simulink model "Blood_platelet_Count_V3"  (R2022a)
settings: Solver=VariableStepAuto  StartTime=0.0  StopTime=10.0  RelTol=1e-3
libraries: simulink x9
settings Model: Creator=KVJ RAMAN  LastModifiedBy=hp

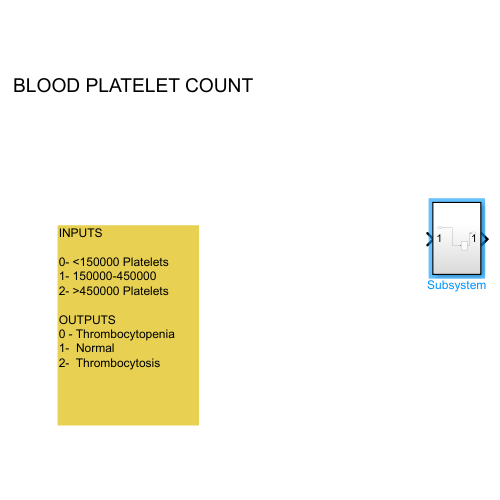
[thumbnail: Simulink's stored preview of the top-level diagram]
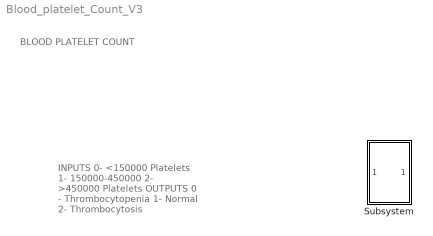
== system Blood_platelet_Count_V3 ==
  note: BLOOD PLATELET COUNT
  note: INPUTS
      |
      | 0- <150000 Platelets
      | 1- 150000-450000
      | 2- >450000 Platelets
      |
      | OUTPUTS
      | 0 - Thrombocytopenia
      | 1-  Normal
      | 2-  Thrombocytosis
  Subsystem : Subsystem

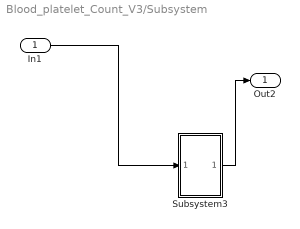
== system Blood_platelet_Count_V3/Subsystem ==
  In1 : Inport
  Subsystem3 : Subsystem
  Out2 : Outport
  wires:
  In1/1 -> Subsystem3/1(In1)
  Subsystem3/1(Out2) -> Out2/1

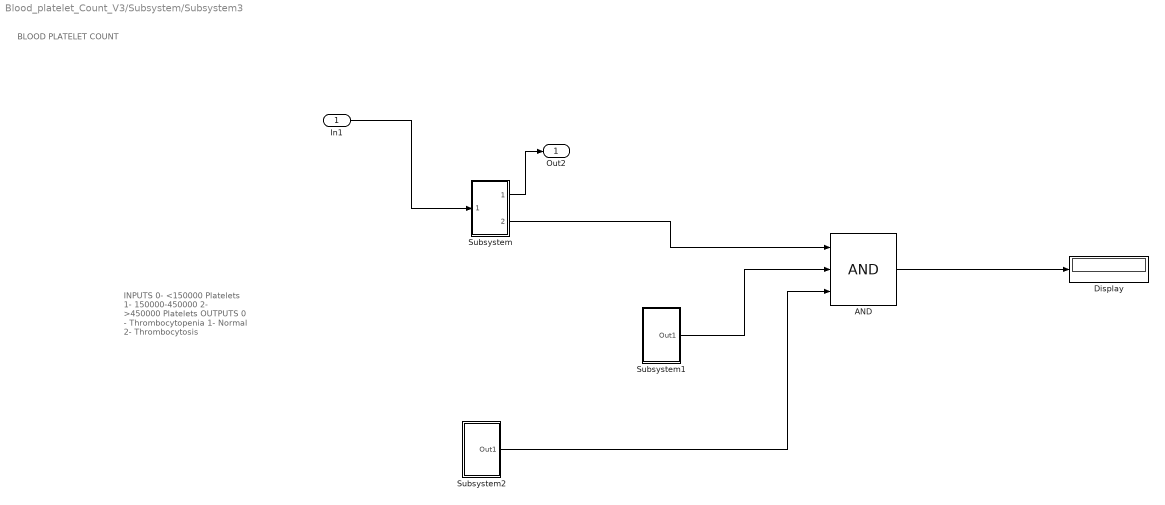
== system Blood_platelet_Count_V3/Subsystem/Subsystem3 ==
  note: BLOOD PLATELET COUNT
  note: INPUTS
      |
      | 0- <150000 Platelets
      | 1- 150000-450000
      | 2- >450000 Platelets
      |
      | OUTPUTS
      | 0 - Thrombocytopenia
      | 1-  Normal
      | 2-  Thrombocytosis
  In1 : Inport
  AND : Logic  Inputs=3  IconShape=distinctive  AllPortsSameDT=off  OutDataTypeStr=boolean
  Display : Display
  Subsystem : Subsystem
  Subsystem1 : Subsystem
  Subsystem2 : Subsystem
  Out2 : Outport
  wires:
  Subsystem2/1(Out1) -> AND/3
  AND/1 -> Display/1
  Subsystem/1(Out2) -> Out2/1
  Subsystem/2(Out1) -> AND/1
  Subsystem1/1(Out1) -> AND/2
  In1/1 -> Subsystem/1(In1)

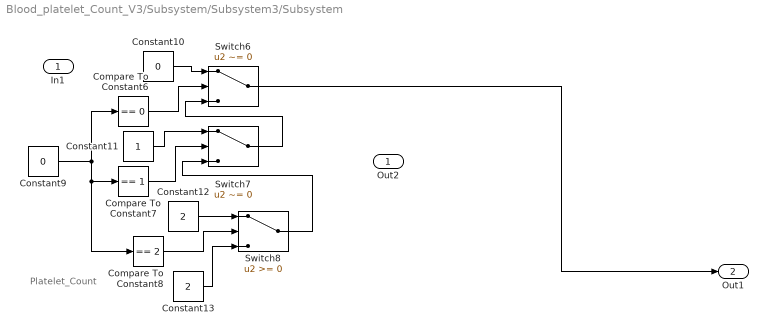
== system Blood_platelet_Count_V3/Subsystem/Subsystem3/Subsystem ==
  note: Platelet_Count
  In1 : Inport
  Compare To Constant6 : simulink/Logic and Bit Operations/Compare To Constant  relop===  const=0  OutDataTypeStr=boolean
  Compare To Constant7 : simulink/Logic and Bit Operations/Compare To Constant  relop===  const=1  OutDataTypeStr=boolean
  Compare To Constant8 : simulink/Logic and Bit Operations/Compare To Constant  relop===  const=2  OutDataTypeStr=boolean
  Constant10 : Constant  Value=0
  Constant11 : Constant
  Constant12 : Constant  Value=2
  Constant13 : Constant  Value=2
  Constant9 : Constant  Value=0
  Switch6 : Switch  Criteria=u2 ~= 0  SaturateOnIntegerOverflow=off  InputSameDT=off
  Switch7 : Switch  Criteria=u2 ~= 0  SaturateOnIntegerOverflow=off  InputSameDT=off
  Switch8 : Switch  SaturateOnIntegerOverflow=off  InputSameDT=off
  Out2 : Outport
  Out1 : Outport  Port=2
  wires:
  Constant11/1 -> Switch7/1
  Compare To Constant6/1 -> Switch6/2
  Switch6/1 -> Out1/1
  Constant9/1 -> Compare To Constant6/1, Compare To Constant8/1, Compare To Constant7/1
  Switch8/1 -> Switch7/3
  Constant10/1 -> Switch6/1
  Compare To Constant7/1 -> Switch7/2
  Switch7/1 -> Switch6/3
  Constant13/1 -> Switch8/3
  Constant12/1 -> Switch8/1
  Compare To Constant8/1 -> Switch8/2

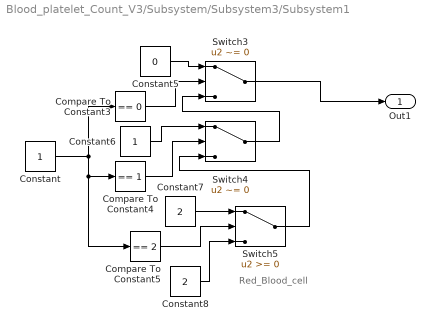
== system Blood_platelet_Count_V3/Subsystem/Subsystem3/Subsystem1 ==
  note: Red_Blood_cell
  Compare To Constant3 : simulink/Logic and Bit Operations/Compare To Constant  relop===  const=0  OutDataTypeStr=boolean
  Compare To Constant4 : simulink/Logic and Bit Operations/Compare To Constant  relop===  const=1  OutDataTypeStr=boolean
  Compare To Constant5 : simulink/Logic and Bit Operations/Compare To Constant  relop===  const=2  OutDataTypeStr=boolean
  Constant : Constant
  Constant5 : Constant  Value=0
  Constant6 : Constant
  Constant7 : Constant  Value=2
  Constant8 : Constant  Value=2
  Switch3 : Switch  Criteria=u2 ~= 0  SaturateOnIntegerOverflow=off  InputSameDT=off
  Switch4 : Switch  Criteria=u2 ~= 0  SaturateOnIntegerOverflow=off  InputSameDT=off
  Switch5 : Switch  SaturateOnIntegerOverflow=off  InputSameDT=off
  Out1 : Outport
  wires:
  Switch4/1 -> Switch3/3
  Compare To Constant4/1 -> Switch4/2
  Constant6/1 -> Switch4/1
  Switch5/1 -> Switch4/3
  Constant5/1 -> Switch3/1
  Constant8/1 -> Switch5/3
  Compare To Constant5/1 -> Switch5/2
  Constant7/1 -> Switch5/1
  Compare To Constant3/1 -> Switch3/2
  Constant/1 -> Compare To Constant3/1, Compare To Constant5/1, Compare To Constant4/1
  Switch3/1 -> Out1/1

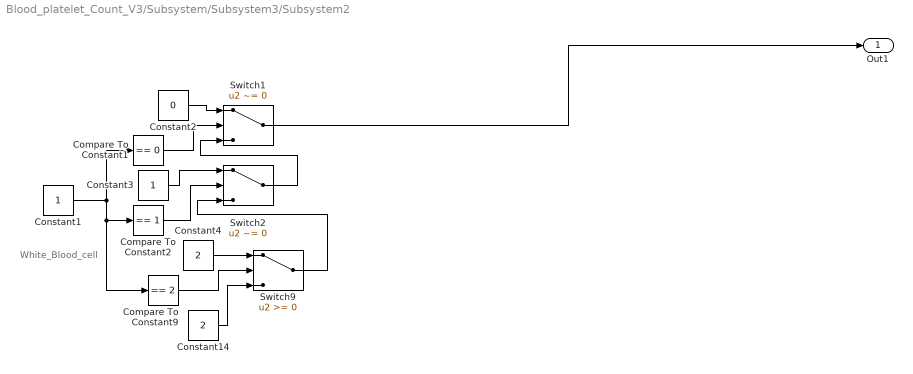
== system Blood_platelet_Count_V3/Subsystem/Subsystem3/Subsystem2 ==
  note: White_Blood_cell
  Compare To Constant1 : simulink/Logic and Bit Operations/Compare To Constant  relop===  const=0  OutDataTypeStr=boolean
  Compare To Constant2 : simulink/Logic and Bit Operations/Compare To Constant  relop===  const=1  OutDataTypeStr=boolean
  Compare To Constant9 : simulink/Logic and Bit Operations/Compare To Constant  relop===  const=2  OutDataTypeStr=boolean
  Constant1 : Constant
  Constant14 : Constant  Value=2
  Constant2 : Constant  Value=0
  Constant3 : Constant
  Constant4 : Constant  Value=2
  Switch1 : Switch  Criteria=u2 ~= 0  SaturateOnIntegerOverflow=off  InputSameDT=off
  Switch2 : Switch  Criteria=u2 ~= 0  SaturateOnIntegerOverflow=off  InputSameDT=off
  Switch9 : Switch  SaturateOnIntegerOverflow=off  InputSameDT=off
  Out1 : Outport
  wires:
  Constant1/1 -> Compare To Constant1/1, Compare To Constant9/1, Compare To Constant2/1
  Compare To Constant9/1 -> Switch9/2
  Switch9/1 -> Switch2/3
  Constant14/1 -> Switch9/3
  Constant2/1 -> Switch1/1
  Constant4/1 -> Switch9/1
  Compare To Constant1/1 -> Switch1/2
  Constant3/1 -> Switch2/1
  Switch2/1 -> Switch1/3
  Compare To Constant2/1 -> Switch2/2
  Switch1/1 -> Out1/1
